simulink model "MBD_problem_3"  (R2020b)
settings: Solver=VariableStepAuto  StartTime=0.0  StopTime=50  RelTol=1e-3
settings Model: Creator=Lenovo  LastModifiedBy=Lenovo
settings DataIOCC: ExternalInput=[t, noise]  LoadExternalInput=on  SaveFormat=Array  ReturnWorkspaceOutputs=off

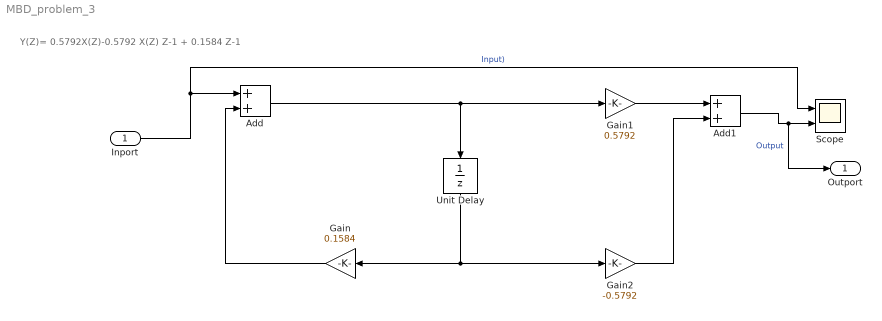
== system MBD_problem_3 ==
  note: Y(Z)= 0.5792X(Z)-0.5792 X(Z) Z-1 + 0.1584 Z-1
  Inport : Inport
  Add : Sum
  Add1 : Sum
  Gain : Gain  Gain=0.1584
  Gain1 : Gain  Gain=0.5792
  Gain2 : Gain  Gain=-0.5792
  Scope : Scope  NumInputPorts=2
  Unit Delay : UnitDelay  SampleTime=-1  HasFrameUpgradeWarning=on
  Outport : Outport
  wires:
  Inport/1 -> Scope/1, Add/1  "Input)"
  Add/1 -> Unit Delay/1, Gain1/1
  Gain/1 -> Add/2
  Unit Delay/1 -> Gain2/1, Gain/1
  Gain1/1 -> Add1/1
  Gain2/1 -> Add1/2
  Add1/1 -> Outport/1, Scope/2  "Output"
